simulink model "Commande_RoueGauche_Reel"  (R2015a)
settings: Solver=ode3  StartTime=0.0  StopTime=inf  RelTol=1e-3
InitFcn:
  | load('LeftInput_Measures.mat');
  | load('LeftOutput_Measures.mat');
  | Parametres_Rover
undefined symbols (not defined in the file): DL, EncRes, IL, NL, PL, rL, RroueL
libraries: simulink x1, Wheels x1
settings Model: SimulationMode=external  ExtModeTrigDuration=2  Creator=tbaroche  LastModifiedBy=tbaroche
settings OptimizationCC: OptimizeModelRefInitCode=on  LifeSpan=1
settings DebuggingCC: UnderspecifiedInitializationDetection=Classic  MergeDetectMultiDrivingBlocksExec=none
settings HardwareCC: ProdLargestAtomicInteger=Long  ProdLargestAtomicFloat=Double  ProdEndianess=LittleEndian  ProdHWDeviceType=ARM Compatible->ARM Cortex
settings RTWCC: SystemTargetFile=realtime.tlc  GenerateMakefile=off  TemplateMakefile=realtime.tmf  Description=Run on Target Hardware  RTWVerbose=off
settings ERTTargetCC: CombineOutputUpdateFcns=off  ExtModeTransport=3  ExtModeMexFile=ext_serial_win32_comm_rtt  ExtModeMexArgs=0 1 9600  ERTSrcFileBannerTemplate=realtime_code_template.cgt  ERTHdrFileBannerTemplate=realtime_code_template.cgt  ERTDataSrcFileTemplate=realtime_code_template.cgt  ERTDataHdrFileTemplate=realtime_code_template.cgt  ERTCustomFileTemplate=realtime_file_process.tlc

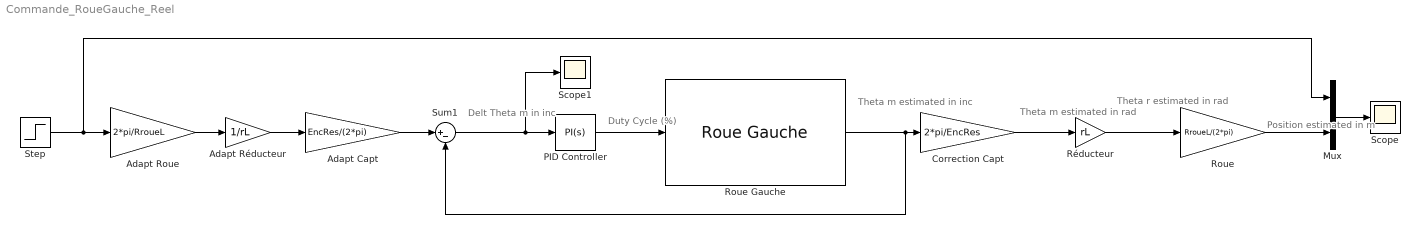
== system Commande_RoueGauche_Reel ==
  note: Position
      | estimated
      | in m
  note: Theta m
      | estimated
      | in inc
  note: Theta r
      | estimated
      | in rad
  note: Theta m
      | estimated
      | in rad
  note: Duty Cycle
      |  (%)
  note: Delt Theta m
      | in inc
  Adapt Roue : Gain  Gain=2*pi/RroueL  ParamDataTypeStr=double
  Adapt Réducteur : Gain  Gain=1/rL
  Adapt Capt : Gain  Gain=EncRes/(2*pi)
  Correction Capt : Gain  Gain=2*pi/EncRes
  Mux : Mux  Inputs=2
  PID Controller : simulink/Continuous/PID Controller  Controller=PI  TimeDomain=Continuous-time  SampleTime=-1  IntegratorMethod=Forward Euler  FilterMethod=Forward Euler  Form=Parallel  UseFilter=on  ControllerParametersSource=internal  P=PL  I=IL  D=DL  N=NL  InitialConditionSource=internal  InitialConditionForIntegrator=0  InitialConditionForFilter=0  ExternalReset=none  LimitOutput=off  UpperSaturationLimit=inf  LowerSaturationLimit=-inf  LinearizeAsGain=on  AntiWindupMode=none  Kb=1  TrackingMode=off  Kt=1  PParamMin=[]  PParamMax=[]  IParamMin=[]  IParamMax=[]  DParamMin=[]  DParamMax=[]  NParamMin=[]  NParamMax=[]  KbParamMin=[]  KbParamMax=[]  KtParamMin=[]  KtParamMax=[]  POutMin=[]  POutMax=[]  IOutMin=[]  IOutMax=[]  DOutMin=[]  DOutMax=[]  NOutMin=[]  NOutMax=[]  KbOutMin=[]  KbOutMax=[]  KtOutMin=[]  KtOutMax=[]  IntegratorOutMin=[]  IntegratorOutMax=[]  FilterOutMin=[]  FilterOutMax=[]  SumOutMin=[]  SumOutMax=[]  SumI1OutMin=[]  SumI1OutMax=[]  SumI2OutMin=[]  SumI2OutMax=[]  SumI3OutMin=[]  SumI3OutMax=[]  SumDOutMin=[]  SumDOutMax=[]  SaturationOutMin=[]  SaturationOutMax=[]  IntegratorContinuousStateAttributes=''  IntegratorStateMustResolveToSignalObject=off  IntegratorRTWStateStorageClass=Auto  FilterContinuousStateAttributes=''  FilterStateMustResolveToSignalObject=off  FilterRTWStateStorageClass=Auto  DifferentiatorICPrevScaledInput=0  DifferentiatorOutMin=[]  DifferentiatorOutMax=[]
  Roue : Gain  Gain=RroueL/(2*pi)  ParamDataTypeStr=double
  Roue Gauche : Wheels/Roue Gauche
  Réducteur : Gain  Gain=rL
  Scope : Scope
      settings: YMin=0.01575  YMax=0.02025
  Scope1 : Scope
      settings: YMin=-250  YMax=2500
  Step : Step  Time=0  After=0.005  SampleTime=0
  Sum1 : Sum  Inputs=|+-
  wires:
  PID Controller/1 -> Roue Gauche/1
  Sum1/1 -> Scope1/1, PID Controller/1
  Correction Capt/1 -> Réducteur/1
  Réducteur/1 -> Roue/1
  Roue/1 -> Mux/2
  Mux/1 -> Scope/1
  Roue Gauche/1 -> Correction Capt/1, Sum1/2
  Adapt Capt/1 -> Sum1/1
  Adapt Réducteur/1 -> Adapt Capt/1
  Adapt Roue/1 -> Adapt Réducteur/1
  Step/1 -> Mux/1, Adapt Roue/1
